simulink model "untitled"  (R2019b)
settings: Solver=VariableStepAuto  StartTime=0.0  StopTime=50  RelTol=1e-3
undefined symbols (not defined in the file or in its folder): sigbuilder_block
libraries: simulink x4
settings Model: EnablePacing=on  Creator=YJR  LastModifiedBy=YJR

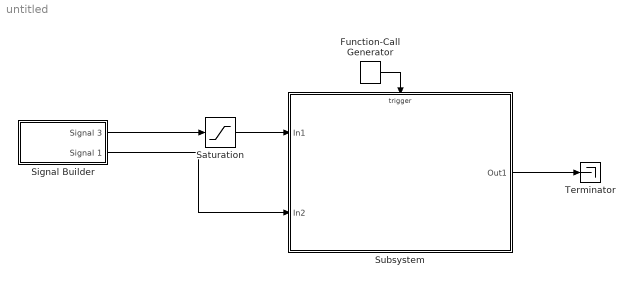
== system untitled ==
  Function-Call Generator : simulink/Ports & Subsystems/Function-Call Generator  sample_time=0.01  numberOfIterations=1
  Saturation : Saturate  UpperLimit=inf  LowerLimit=0
  Signal Builder : Subsystem  Tag=STV Subsys  LoadFcn=sigbuilder_block('load');  StartFcn=sigbuilder_block('start');  StopFcn=sigbuilder_block('stop');  ClipboardFcn=sigbuilder_block('clipboard');  mask(Sigbuilder block){tuvar=[0:10]}
      mask help: Simulink:masks:SigbuilderBlock_MD
      mask init:
      | if ~strcmp(get_param(bdroot(gcbh),'SimulationStatus'),'stopped') tuvar = sigbuilder_block('maskInit'); end
      settings: CopyFcn=sigbuilder_block('copy');  DeleteFcn=sigbuilder_block('delete');  ModelCloseFcn=sigbuilder_block('modelClose');  PreSaveFcn=sigbuilder_block('preSave');  PauseFcn=sigbuilder_block('pause');  ContinueFcn=sigbuilder_block('continue');  NameChangeFcn=sigbuilder_block('namechange');  OpenFcn=sigbuilder_block('open',[5.4 36 1141.2 517.8 ]);  CloseFcn=sigbuilder_block('close');
      mask Display: plot(0, 0, 100, 100,[2, 2, 32, 32, 2], [68, 8, 8, 68, 68],[32, 2], [38, 38], [32, 19, 2],[53, 60, 44], [32, 17, 17, 2],[16, 16, 31, 31]);txt = getActiveGroup(gcbh);text(2, 100, txt,'verticalAlignment', 'top');
  Subsystem : Subsystem
  Terminator : Terminator
  wires:
  Signal Builder/1(Signal 3) -> Saturation/1
  Function-Call Generator/1 -> Subsystem/Trigger
  Subsystem/1(Out1) -> Terminator/1
  Signal Builder/2(Signal 1) -> Subsystem/2(In2)
  Saturation/1 -> Subsystem/1(In1)

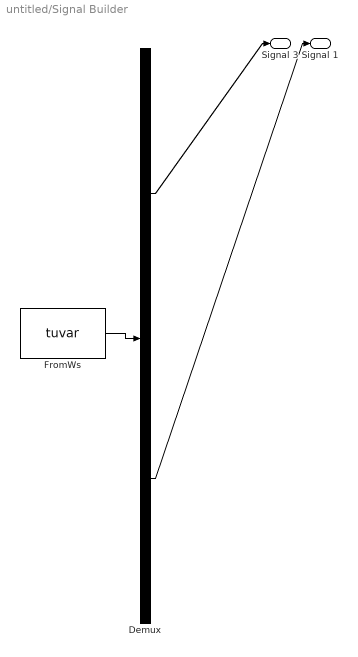
== system untitled/Signal Builder ==
  Demux : Demux  Tag=STV Demux  Outputs=2
  FromWs : FromWorkspace  Tag=STV FromWs  VariableName=tuvar  SampleTime=0
      SigBuilderData=|
      | common.afterFinalStr = 'Extrapolate'
      | common.sampleTime = 0
      | dataSet.timeRange = [0 50]
      | dataSet.name = 'Group 1'
      | sbobj.Groups.Name = 'Group 1'
      | sbobj.Groups.Signals(1).Name = 'Signal 3'
      | sbobj.Groups.Signals(1).XData = [0 5 20 30 30 50]
      | sbobj.Groups.Signals(1).YData = [0 0 500 500 0 0]
      | sbobj.Groups.Signals(2).Name = 'Signal 1'
      | sbobj.Groups.Signals(2).XData = [0 4.9 4.9 6 6 50]
      | sbobj.Groups.Signals(2).YData = [0 0 1 1 0 0]
      | sbobj.Groups.TimeRange = [0 50]
  Signal 3 : Outport  Tag=STV Outport
  Signal 1 : Outport  Tag=STV Outport  Port=2
  wires:
  FromWs/1 -> Demux/1
  Demux/1 -> Signal 3/1
  Demux/2 -> Signal 1/1

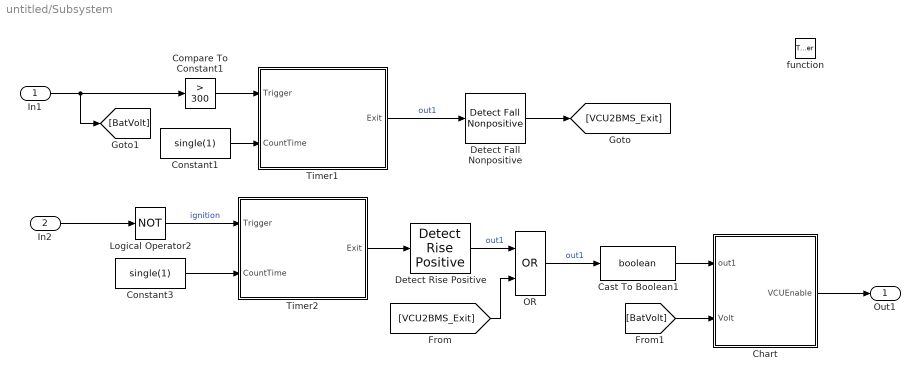
== system untitled/Subsystem ==
  In1 : Inport
  In2 : Inport  Port=2
  function : TriggerPort  TriggerType=function-call  VariantControl=Variant
  Cast To Boolean1 : DataTypeConversion  OutDataTypeStr=boolean
  Chart : Stateflow chart  BlockKeywords=__PRM__SERIALIZED__DATA__:Stateflow Chart,Stateflow Diagram  TreatAsAtomicUnit=on
  Compare To Constant1 : simulink/Logic and Bit Operations/Compare To Constant  relop=>  const=300  OutDataTypeStr=boolean
  Constant1 : Constant  Value=single(1)
  Constant3 : Constant  Value=single(1)
  Detect Fall Nonpositive : simulink/Logic and Bit Operations/Detect Fall Nonpositive  vinit=1  OutDataTypeStr=boolean
      settings: SourceProductName=Simulink  SourceProductBaseCode=SL
  Detect Rise Positive : simulink/Logic and Bit Operations/Detect Rise Positive  vinit=0  OutDataTypeStr=boolean
  Logical Operator2 : Logic  Operator=NOT  AllPortsSameDT=off  OutDataTypeStr=boolean
  OR : Logic  Operator=OR  AllPortsSameDT=off  OutDataTypeStr=boolean
  Timer1 : Stateflow chart  TreatAsAtomicUnit=on
  Timer2 : Stateflow chart  TreatAsAtomicUnit=on
  Out1 : Outport
  wires:
  OR/1 -> Cast To Boolean1/1  "out1"
  Timer1/1(Exit) -> Detect Fall Nonpositive/1  "out1"
  Detect Fall Nonpositive/1 -> [VCU2BMS_Exit]
  [VCU2BMS_Exit] -> OR/2
  Detect Rise Positive/1 -> OR/1  "out1"
  Timer2/1(Exit) -> Detect Rise Positive/1
  Constant3/1 -> Timer2/2(CountTime)
  In1/1 -> [BatVolt], Compare To Constant1/1
  Constant1/1 -> Timer1/2(CountTime)
  Compare To Constant1/1 -> Timer1/1(Trigger)
  Logical Operator2/1 -> Timer2/1(Trigger)  "ignition"
  In2/1 -> Logical Operator2/1
  Chart/1(VCUEnable) -> Out1/1
  Cast To Boolean1/1 -> Chart/1(out1)
  [BatVolt] -> Chart/2(Volt)

== stateflow chart untitled/Subsystem/Timer1 ==
  state Trigger
    en:
    x = x + 0.01;
    Exit=0;
  state Out
    en:
    Exit=1;
    x=0;
  state InterState
    en:
    x=0;
  Trigger -> Trigger [order 1] : [Trigger&&x<CountTime]
  Trigger -> Out [order 2] : [x>=CountTime]
  (default) -> Trigger
  Out -> Trigger : [~Trigger]
  InterState -> Trigger : [Trigger]
  Trigger -> InterState [order 3] : [x<CountTime&&~Trigger]
  data: Trigger input; CountTime input; Exit output; x local =0

== stateflow chart untitled/Subsystem/Chart ==
  state STATEON
    state initstate
      en:
      VCUEnable=false;
    state ON
      en:
      VCUEnable=true;
    (default) -> initstate
    initstate -> ON : after(0.2,sec)[out1]
  state STATEOFF
    state initstate1
      en:
      VCUEnable=true;
    state OFF
      en:
      VCUEnable=false;
    (default) -> initstate1
    initstate1 -> OFF : after(0.2,sec)[out1]
  (default) -> STATEON
  STATEOFF -> STATEON : after(10,sec)[Volt<400]
  ON -> STATEOFF
  OFF -> STATEON
  data: out1 input boolean; VCUEnable output boolean; Volt input

== stateflow chart untitled/Subsystem/Timer2 ==
  state Trigger
    en:
    x = x + 0.01;
    Exit=0;
  state Out
    en:
    Exit=1;
    x=0;
  state InterState
    en:
    x=0;
  Trigger -> Trigger [order 1] : [Trigger&&x<CountTime]
  Trigger -> Out [order 2] : [x>=CountTime]
  (default) -> Trigger
  Out -> Trigger : [~Trigger]
  InterState -> Trigger : [Trigger]
  Trigger -> InterState [order 3] : [x<CountTime&&~Trigger]
  data: Trigger input; CountTime input; Exit output; x local =0
